simulink model "Q1"  (R2018b)
settings: Solver=VariableStepAuto  StartTime=0.0  StopTime=500  RelTol=1e-3
undefined symbols (not defined in the file): m, n
settings Model: Creator=lenovo  LastModifiedBy=lenovo

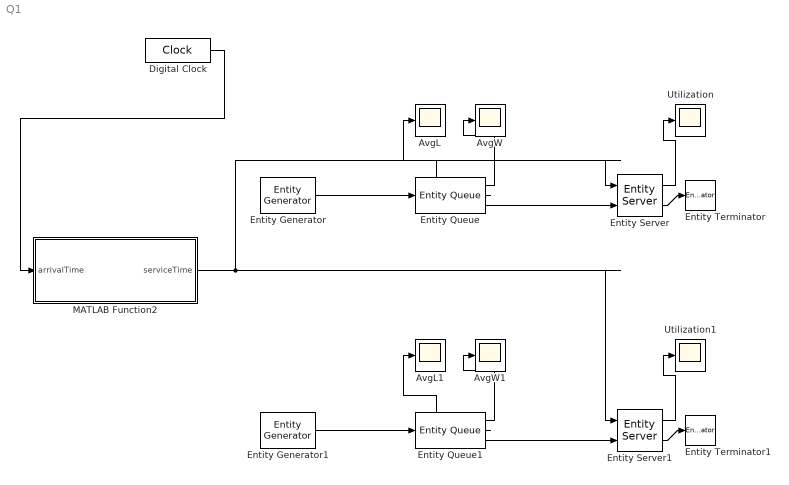
== system Q1 ==
  AvgL : Scope
  AvgL1 : Scope
  AvgW : Scope
  AvgW1 : Scope
  Digital Clock : DigitalClock  SampleTime=1000
  Entity Generator : EntityGenerator  OutputPortMessageModes=m  TimeSource=MATLAB action  IntergenerationTimeAction=|  EntityType=Structured  EntityTypeName=Entity
      | persistent rngInit;
      | if isempty(rngInit)
      |     seed = 12345;
      |     rng(seed);
      |     rngInit = true;
      | end
      | 
      | % Pattern: Exponential distribution
      | mu = 1.8;
      | dt = -mu * log(1 - rand());
  Entity Generator1 : EntityGenerator  OutputPortMessageModes=m  TimeSource=MATLAB action  IntergenerationTimeAction=|  EntityType=Structured  EntityTypeName=Entity
      | persistent rngInit;
      | if isempty(rngInit)
      |     seed = 12345;
      |     rng(seed);
      |     rngInit = true;
      | end
      | 
      | % Pattern: Exponential distribution
      | mu = 1.8;
      | dt = -mu * log(1 - rand());
  Entity Queue : EntityQueue  InputPortMessageModes=m  OutputPortMessageModes=n,n,m  Capacity=inf  AverageWait=on  AverageQueueLength=on
      settings: OutputPortMap=o2,o3,o5
  Entity Queue1 : EntityQueue  InputPortMessageModes=m  OutputPortMessageModes=n,n,m  Capacity=inf  QueueType=LIFO  AverageWait=on  AverageQueueLength=on
      settings: OutputPortMap=o2,o3,o5
  Entity Server : EntityServer  InputPortMessageModes=n,m  OutputPortMessageModes=n,m  Capacity=1  ServiceTimeSource=Signal port  ServiceTimeAttributeName=entity  ServiceTimeAction=|  Utilization=on
      | SimClk = get_currentTime('Q1');
      | if SimClk < 100
      |     dt = -1*log(1-rand());
      | elseif SimClk < 200
      |     dt = -2*log(1-rand());
      | elseif SimClk < 300
      |     dt = -4*log(1-rand());
      | elseif SimClk < 400
      |     dt = -8*log(1-rand());
      | else
      |     dt = -10*log(1-rand());
      | end
      settings: InputPortMap=u0,u2  OutputPortMap=o5,o9
  Entity Server1 : EntityServer  InputPortMessageModes=n,m  OutputPortMessageModes=n,m  Capacity=1  ServiceTimeSource=Signal port  ServiceTimeAttributeName=entity  ServiceTimeAction=dt = entity.Attribute1;  Utilization=on
      settings: InputPortMap=u0,u2  OutputPortMap=o5,o9
  Entity Terminator : EntityTerminator  InputPortMessageModes=m
  Entity Terminator1 : EntityTerminator  InputPortMessageModes=m
  MATLAB Function2 : MATLAB Function  TreatAsAtomicUnit=on
  Utilization : Scope
  Utilization1 : Scope
  wires:
  Entity Queue/3 -> Entity Server/2
  Entity Generator/1 -> Entity Queue/1
  Entity Server/2 -> Entity Terminator/1
  Entity Server/1 -> Utilization/1
  Entity Queue/1 -> AvgW/1
  Entity Queue/2 -> AvgL/1
  Entity Server1/2 -> Entity Terminator1/1
  Entity Queue1/3 -> Entity Server1/2
  Entity Server1/1 -> Utilization1/1
  Entity Queue1/2 -> AvgL1/1
  Entity Generator1/1 -> Entity Queue1/1
  Entity Queue1/1 -> AvgW1/1
  Digital Clock/1 -> MATLAB Function2/1(arrivalTime)
  MATLAB Function2/1(serviceTime) -> Entity Server1/1, Entity Server/1

== matlab function Q1/MATLAB Function2 ==
  data: arrivalTime input; serviceTime output
function serviceTime = ST_function(arrivalTime)
    if arrivalTime < 100
         serviceTime = -1*log(1-rand());
    elseif arrivalTime >= 100 && arrivalTime < 200
         serviceTime = -3*log(1-rand());
    elseif arrivalTime >= 200 && arrivalTime < 300
         serviceTime = -9*log(1-rand());
    elseif arrivalTime >= 300 && arrivalTime < 400
         serviceTime = -27*log(1-rand());
    else
         serviceTime = -81*log(1-rand());
    end
